simulink model "MultirotorSimPx4SeparateRotors"  (R2016b)
settings: Solver=VariableStepAuto  StartTime=0.0  StopTime=Simulation.T_END  MaxStep=Simulation.TS_MAX  RelTol=1e-3  EnableMultiTasking=on
PreLoadFcn:
  | % InitializeParameters;
undefined symbols (not defined in the file): Initial
libraries: Px4Library x19, QuaternionLibrary x12, simulink_extras x6
settings Model: Creator=jban039  LastModifiedBy=jeremie
settings DataIOCC: Decimation=10  ReturnWorkspaceOutputs=on  OutputOption=SpecifiedOutputTimes  OutputTimes=Simulation.T_OUT
settings OptimizationCC: LifeSpan=inf
settings DebuggingCC: ReadBeforeWriteMsg=DisableAll  WriteAfterWriteMsg=DisableAll  WriteAfterReadMsg=DisableAll  MultiTaskDSMMsg=none  UnconnectedLineMsg=none  AllowSymbolicDim=off  SFUnexpectedBacktrackingDiag=warning  SFNoUnconditionalDefaultTransitionDiag=warning  SFExecutionAtInitializationDiag=none
settings ModelReferenceCC: UpdateModelReferenceTargets=IfOutOfDate  ModelReferenceMinAlgLoopOccurrences=on  PropagateSignalLabelsOutOfModel=off
settings SFSimCC: SFSimEcho=off
settings GRTTargetCC: TargetLangStandard=C89/C90 (ANSI)
settings ConfigComp: CovMetricSettings=dw  CovHtmlReporting=on  CovSaveCumulativeToWorkspaceVar=on  CovSaveSingleToWorkspaceVar=on  CovExternalEMLEnable=off

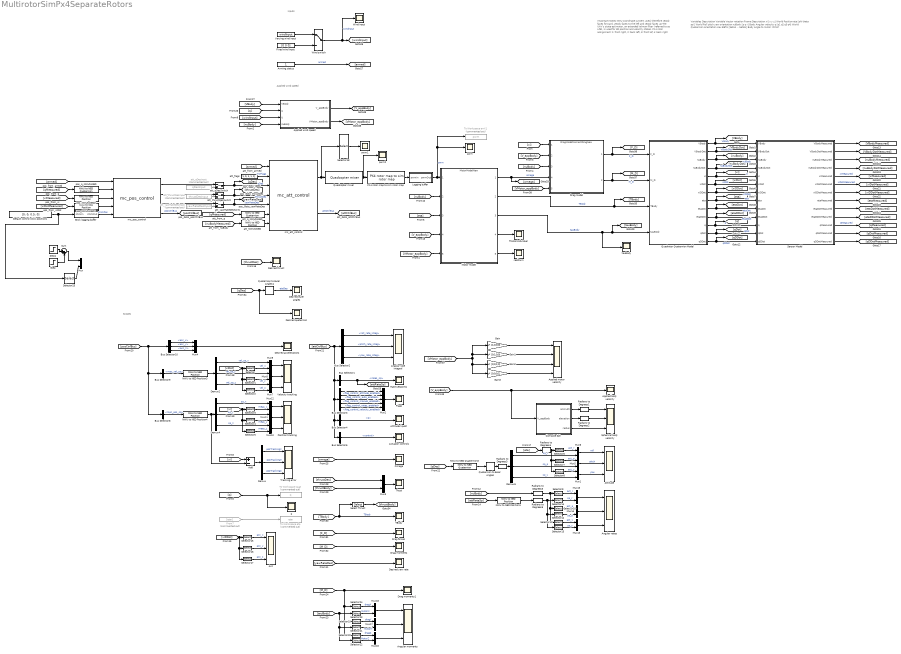
== system MultirotorSimPx4SeparateRotors ==
  note: Important Notes
      |
      | NWU coordinate system used, therefore xBody faces forward, yBody faces to the left and xBody faces up
      | The UAV's state estimator, an extended kalman filter (referred to as LPE), is used for 3D position and velocity states.
      | PX4 rotor assignment: 1: front right, 2: back left, 3: front lef, 4: back right
  note: Variables Description
      |
      | Variable
      | Vector notation
      | Frame
      | Description
      |
      | xi
      | [x y z]
      | World
      | Position
      |
      | eta
      | [phi theta psi]
      | World
      | Roll pitch yaw orientation
      |
      | nuBody
      | [p q r]
      | Body
      | Angular velocity
      |
      | q
      | [q1 q2 q3 q4]
      | World
      | Quaternion orientation
      |
      | Uav.BETA
      | [beta1 ... betaN]
      | Body
      | Angle to motor (CCW)
  note: Applied wind speed
  note: Inputs
  note: Scopes
  Acc : Scope  NumInputPorts=3
  Actuator controls : Scope
  Add : Sum  Inputs=+-
  Angular moments : Scope  NumInputPorts=3
  Angular rate integral : Scope  NumInputPorts=3
  Angular rates : Scope  NumInputPorts=3
  Applied body velocity : Scope
  Applied motor velocity : Scope  NumInputPorts=4
  Applied wind speed : Subsystem
  Arming status : Constant
  Attitude : Scope  NumInputPorts=3
  Attitude (quat) : Scope
  Bus Selector1 : BusSelector  OutputSignals=rates_sp
  Bus Selector10 : BusSelector  OutputSignals=mpc_local_pos_sp.acc_x,mpc_local_pos_sp.acc_y,mpc_local_pos_sp.acc_z
  Bus Selector2 : BusSelector  OutputSignals=controller_status.roll_rate_integ,controller_status.pitch_rate_integ,controller_status.yaw_rate_integ
  Bus Selector3 : BusSelector  OutputSignals=v_control_mode.flag_control_attitude_enabled,v_control_mode.flag_control_auto_enabled,v_control_mode.flag_control_manual_enabled,v_control_mode.flag_control_rates_enabled,v_control_mode.flag_control_velocity_enabled
  Bus Selector4 : BusSelector  OutputSignals=ctrl_state.q
  Bus Selector6 : BusSelector  OutputSignals=actuators.control
  Bus Selector8 : BusSelector  OutputSignals=mpc_pos_sp
  Bus Selector9 : BusSelector  OutputSignals=mpc_vel_sp
  Compute Sph : MATLAB Function  TreatAsAtomicUnit=on
  Default control stick positions : Constant  Value=[0; 0; 0.5; 0]
  Demux{,2,4,6} (4 alike) : Demux  Outputs=3
  Desired accelerations : Scope
  Desired euler angles : Scope
  Desired quaternion : Scope
  Desired thrust : Scope
  Desired yaw rate : Scope
  Drag forces : Scope
  Drag model : ModelReference  ModelNameDialog=DragModelMomentDragNew  SimulationMode=Normal  ModelReferenceVersion=1.250
  Drag moments : Scope
  Drag moments1 : Scope
  Fixed wind input : Constant  Value=[0 0 0]
  Flags : Scope
  From7 : From  Commented=on  GotoTag=eta
  Gain : Gain  Gain=[1;0;0;0]  Multiplication=Matrix(u*K)
  Gain1 : Gain  Gain=[0;1;0;0]  Multiplication=Matrix(u*K)
  Gain2 : Gain  Gain=[0;0;1;0]  Multiplication=Matrix(u*K)
  Gain3 : Gain  Gain=[0;0;0;1]  Multiplication=Matrix(u*K)
  Logging buffer : Subsystem
  Motor model : ModelReference  ModelNameDialog=MotorModelNew  SimulationMode=Normal  ModelReferenceVersion=1.289
  Mux{,1,3,5..18} (17 alike) : Mux  Inputs=2
  Mux2 : Mux  Inputs=5
  Mux4 : Mux  Inputs=3
  NWU to NED Position1 : Px4Library/NWU to NED Position
  NWU to NED Position3 : Px4Library/NWU to NED Position
  NWU to NED Position4 : Px4Library/NWU to NED Position
  NWU to NED Quaternion3 : Px4Library/NWU to NED Quaternion
  Omega : Scope
  PX4 rotor map to sim rotor map : Px4Library/PX4 rotor map to sim rotor map  SystemSampleTime=-1
  Position tracking : Scope  NumInputPorts=3
  Quadcopter mixer : Px4Library/Quadcopter mixer  MC_SAMPLING_PERIOD=0.002
  Quadrotor Quaternion Model : Subsystem
  Quaternion to Euler Angles : QuaternionLibrary/Quaternion to Euler Angles
  Quaternion to Euler Angles1 : QuaternionLibrary/Quaternion to Euler Angles
  Radians to Degrees{1..6} (6 alike) : simulink_extras/Transformations/Radians to Degrees
  Rate setpoints : Scope
  Select Thrust : Selector  InputPortWidth=3  IndexOptions=Index vector (dialog)  Indices=[3]  OutputSizes=1
  Selector{,3,6,9,14..15,23..24} (8 alike) : Selector  InputPortWidth=3  IndexOptions=Index vector (dialog)  Indices=1  OutputSizes=1
  Selector{1,4,7,10,12,16,19,21} (8 alike) : Selector  InputPortWidth=3  IndexOptions=Index vector (dialog)  Indices=2  OutputSizes=1
  Selector{2,5,8,11,13,17,20,22} (8 alike) : Selector  InputPortWidth=3  IndexOptions=Index vector (dialog)  Indices=3  OutputSizes=1
  Selector18 : Selector  InputPortWidth=8  IndexOptions=Index vector (dialog)  Indices=[1 2 3]  OutputSizes=1
  Selector25 : Selector  InputPortWidth=4  IndexOptions=Index vector (dialog)  Indices=[ 2 3 4 ]  OutputSizes=1
  Sensor Model : Subsystem
  Spherical body velocity : Scope  NumInputPorts=3
  Step : Step  Time=100  After=0.2  SampleTime=0
  Step1 : Step  Time=105  After=-0.2  SampleTime=0
  Stick logging buffer : Subsystem
  Sum : Sum  Inputs=|++
  TBody : Scope
  TMotorIndividual : Scope
  Thust : Scope
  To Workspace errX1 : ToWorkspace  Commented=on  VariableName=pwm  SampleTime=0.01
      settings: Save2DSignal=2-D array (concatenate along first dimension)
  To Workspace eta : ToWorkspace  Commented=on  VariableName=eta  SaveFormat=Structure With Time  SampleTime=0.01
  To Workspace quat : ToWorkspace  Commented=on  VariableName=q  SaveFormat=Structure With Time  SampleTime=0.01
  Tracking error : Scope  NumInputPorts=3
  Varying wind input : FromWorkspace  VariableName=windInput  SampleTime=0
  Velocity tracking : Scope  NumInputPorts=3
  Wind Input : Scope
  Wind switch : ManualSwitch
  att_NWUtoNED : Px4Library/NWU to NED Position
  att_flags : Constant  Value=[1, 0, 1, 1, 1]
  att_qDesInput : FromWorkspace  Commented=on  VariableName=qDesInput  SampleTime=0  Interpolate=off  OutputAfterFinalValue=Holding final value
  att_qDesSwitch : ManualSwitch
  att_q_NWUtoNED : Px4Library/NWU to NED Quaternion
  att_thrustDesInput : FromWorkspace  Commented=on  VariableName=thrustDesInput  SampleTime=0  Interpolate=off  OutputAfterFinalValue=Holding final value
  att_thrustDesSwitch : ManualSwitch
  att_yawRateDesInput : FromWorkspace  Commented=on  VariableName=yawRateDesInput  SampleTime=0  Interpolate=off  OutputAfterFinalValue=Holding final value
  att_yawRateDesSwitch : ManualSwitch
  mc_att_control : Px4Library/mc_att_control  MC_SAMPLING_PERIOD=0.004  MC_ROLL_TC=0.2  MC_PITCH_TC=0.2  MC_ROLL_P=6.5  MC_ROLLRATE_P=0.15  MC_ROLLRATE_I=0.05  MC_ROLLRATE_D=0.003  MC_ROLLRATE_FF=0.0  MC_PITCH_P=6.5  MC_PITCHRATE_P=0.15  MC_PITCHRATE_I=0.05  MC_PITCHRATE_D=0.003  MC_PITCHRATE_FF=0.0  MC_YAW_P=2.8  MC_YAWRATE_P=0.2  MC_YAWRATE_I=0.1  MC_YAWRATE_D=0.0  MC_YAWRATE_FF=0.0  MC_YAW_FF=0.5  MC_ROLLRATE_MAX=220.0  MC_PITCHRATE_MAX=220.0  MC_YAWRATE_MAX=200.0  MC_YAWRAUTO_MAX=45.0  MC_ACRO_R_MAX=360.0  MC_ACRO_P_MAX=360.0  MC_ACRO_Y_MAX=360.0  MC_RATT_TH=1.0  MC_TPA_BREAK=1.0  MC_TPA_SLOPE=1.0  VT_OPT_RECOV_EN=0.0  VT_WV_YAWR_SCL=0.15  MC_RR_INT_LIM=0.30  MC_PR_INT_LIM=0.30  MC_TPA_BREAK_P=1.0  MC_TPA_BREAK_I=1.0  MC_TPA_BREAK_D=1.0  MC_TPA_RATE_P=0.0  MC_TPA_RATE_I=0.0  MC_TPA_RATE_D=0.0  VT_TYPE=2  MC_BAT_SCALE_EN=0  MC_YR_INT_LIM=0.30
  mc_pos_control : Px4Library/mc_pos_control  THROTTLE_HOVER=Uav.THROTTLE_HOVER  MPC_SAMPLING_PERIOD=0.02  MPC_THR_MIN=0.120  MPC_THR_HOVER=0.500  MPC_ALTCTL_DZ=0.100  MPC_ALTCTL_DY=0.0  MPC_THR_MAX=0.900  MPC_MANTHR_MIN=0.080  MPC_MANTHR_MAX=0.900  MPC_Z_P=1.000  MPC_Z_VEL_P=0.200  MPC_Z_VEL_I=0.020  MPC_Z_VEL_D=0.0  MPC_Z_VEL_MAX_UP=3.0  MPC_Z_VEL_MAX=1.000  MPC_Z_VEL_MAX_DN=1.000  MPC_Z_FF=0.500  MPC_XY_P=0.950  MPC_XY_VEL_P=0.090  MPC_XY_VEL_I=0.020  MPC_XY_VEL_D=0.010  MPC_XY_CRUISE=5.0  MPC_XY_VEL_MAX=8.0  MPC_XY_FF=0.500  MPC_TILTMAX_AIR=45.0  MPC_TILTMAX_LND=12.0  MPC_LAND_SPEED=0.500  MPC_TKO_SPEED=1.500  MPC_MAN_R_MAX=35.0  MPC_MAN_P_MAX=35.0  MPC_MAN_Y_MAX=200.0  MPC_HOLD_XY_DZ=0.100  MPC_HOLD_MAX_XY=0.800  MPC_HOLD_MAX_Z=0.600  MPC_VELD_LP=5.0  MPC_ACC_HOR_MAX=5.0  MPC_ALT_MODE=0.0  MC_YAWRATE_MAX=200.0  MC_YAW_P=2.8  VT_OPT_RECOV_EN=0.0
  pos_NWUtoNED1 : Px4Library/NWU to NED Position
  pos_NWUtoNED2 : Px4Library/NWU to NED Position
  pos_q_NWUtoNED : Px4Library/NWU to NED Quaternion
  pwm : Scope
  pwm1 : Scope
  pwm2 : Scope
  q : Scope
  realPwm : Scope
  tauBody : Scope
  wires:
  Motor model/1 -> [omega], Drag model/4  "omega"
  Motor model/2 -> [TBody], Quadrotor Quaternion Model/3(TBody)  "TBody"
  Drag model/2 -> [M_D], Quadrotor Quaternion Model/2(M_D)  "M_D"
  Quadrotor Quaternion Model/1(VBody) -> Sensor Model/1(VBody), [VBody]  "VBody"
  Quadrotor Quaternion Model/2(VBodyDot) -> Sensor Model/2(VBodyDot), [VBodyDot]  "VBodyDot"
  Quadrotor Quaternion Model/3(nuBody) -> Sensor Model/3(nuBody), [nuBody]  "nuBody"
  Quadrotor Quaternion Model/4(nuBodyDot) -> Sensor Model/4(nuBodyDot), [nuBodyDot]  "nuBodyDot"
  Quadrotor Quaternion Model/5(xi) -> Sensor Model/5(xi), [xi]  "xi"
  Quadrotor Quaternion Model/6(xiDot) -> Sensor Model/6(xiDot), [xiDot]  "xiDot"
  Quadrotor Quaternion Model/7(xiDDot) -> Sensor Model/7(xiDDot), [xiDDot]  "xiDDot"
  Quadrotor Quaternion Model/8(eta) -> Sensor Model/8(eta), [eta]  "eta"
  Quadrotor Quaternion Model/9(etaDot) -> Sensor Model/9(etaDot), [etaDot]  "etaDot"
  Quadrotor Quaternion Model/10(etaDDot) -> Sensor Model/10(etaDDot), [etaDDot]  "etaDDot"
  [V_appBody] -> Drag model/2
  [nuBody] -> Motor model/2
  Quadrotor Quaternion Model/11(q) -> Sensor Model/11(q), [q]  "q"
  Quadrotor Quaternion Model/12(qDot) -> Sensor Model/12(qDot), [qDot]  "qDot"
  Quadrotor Quaternion Model/13(qDDot) -> Sensor Model/13(qDDot), [qDDot]  "qDDot"
  Drag model/1 -> Quadrotor Quaternion Model/1(F_D), [F_D]  "F_D"
  Sensor Model/1(VBodyMeasured) -> [VBodyMeasured]
  Sensor Model/2(VBodyDotMeasured) -> [VBodyDotMeasured]
  Sensor Model/3(nuBodyMeasured) -> [nuBodyMeasured]
  Sensor Model/4(nuBodyDotMeasured) -> [nuBodyDotMeasured]
  Sensor Model/5(xiMeasured) -> [xiMeasured]  "xiMeasured"
  Sensor Model/6(xiDotMeasured) -> [xiDotMeasured]  "xiDotMeasured"
  Sensor Model/7(xiDDotMeasured) -> [xiDDotMeasured]
  Sensor Model/8(etaMeasured) -> [etaMeasured]
  Sensor Model/9(etaDotMeasured) -> [etaDotMeasured]
  Sensor Model/10(etaDDotMeasured) -> [etaDDotMeasured]
  Sensor Model/11(qMeasured) -> [qMeasured]  "qMeasured"
  Sensor Model/12(qDotMeasured) -> [qDotMeasured]
  Sensor Model/13(qDDotMeasured) -> [qDDotMeasured]
  Logging buffer/1(pwmOut) -> To Workspace errX1/1, pwm/1, Motor model/1  "pwm"
  [nuBodyMeasured] -> att_NWUtoNED/1
  Bus Selector2/1 -> Angular rate integral/1  "<roll_rate_integ>"
  Bus Selector2/2 -> Angular rate integral/2  "<pitch_rate_integ>"
  Bus Selector2/3 -> Angular rate integral/3  "<yaw_rate_integ>"
  [attCtrlBus] -> Bus Selector2/1, Bus Selector1/1, Bus Selector6/1, Bus Selector4/1, Bus Selector3/1
  Bus Selector1/1 -> [attRateSp], Rate setpoints/1  "<rates_sp>"
  Bus Selector3/1 -> Mux2/1  "<flag_control_attitude_enabled>"
  Bus Selector3/2 -> Mux2/2  "<flag_control_auto_enabled>"
  Bus Selector3/3 -> Mux2/3  "<flag_control_manual_enabled>"
  Bus Selector3/4 -> Mux2/4  "<flag_control_rates_enabled>"
  Bus Selector3/5 -> Mux2/5  "<flag_control_velocity_enabled>"
  Mux2/1 -> Flags/1
  Bus Selector4/1 -> Attitude (quat)/1  "<q>"
  Bus Selector6/1 -> Actuator controls/1  "<control>"
  mc_pos_control/1 -> att_qDesSwitch/1
  [posCtrlBus] -> Bus Selector10/1, Bus Selector9/1, Bus Selector8/1
  [qMeasured] -> pos_q_NWUtoNED/1
  Stick logging buffer/1(stickOut) -> mc_pos_control/5  "stickPos"
  [qMeasured] -> att_q_NWUtoNED/1
  att_q_NWUtoNED/1 -> mc_att_control/6
  att_NWUtoNED/1 -> mc_att_control/7
  pos_q_NWUtoNED/1 -> mc_pos_control/2
  mc_pos_control/3 -> att_yawRateDesSwitch/1
  mc_pos_control/2 -> att_thrustDesSwitch/1
  Bus Selector9/1 -> NWU to NED Position3/1  "<mpc_vel_sp>"
  pos_NWUtoNED1/1 -> mc_pos_control/4
  pos_NWUtoNED2/1 -> mc_pos_control/3
  [xiMeasured] -> pos_NWUtoNED2/1
  Bus Selector10/1 -> Mux4/1  "<acc_x>"
  Bus Selector10/2 -> Mux4/2  "<acc_y>"
  Bus Selector10/3 -> Mux4/3  "<acc_z>"
  Mux4/1 -> Desired accelerations/1
  Selector6/1 -> Mux6/1  "act_r"
  Selector7/1 -> Mux5/1  "act_p"
  Mux7/1 -> Velocity tracking/3
  Mux8/1 -> Velocity tracking/2
  Mux9/1 -> Velocity tracking/1
  Demux2/1 -> Mux9/1  "vel_sp_x"
  Selector/1 -> Mux9/2  "vel_x"
  Demux2/2 -> Mux8/1  "vel_sp_y"
  Selector1/1 -> Mux8/2  "vel_y"
  Demux2/3 -> Mux7/1  "vel_sp_z"
  Selector2/1 -> Mux7/2  "vel_z"
  Mux10/1 -> Position tracking/3
  Mux11/1 -> Position tracking/2
  Mux12/1 -> Position tracking/1
  Demux4/1 -> Mux12/1  "sp_x"
  Selector3/1 -> Mux12/2  "meas_x"
  Demux4/2 -> Mux11/1  "sp_y"
  Selector4/1 -> Mux11/2  "meas_y"
  Demux4/3 -> Mux10/1  "sp_z"
  Selector5/1 -> Mux10/2  "meas_z"
  Quaternion to Euler Angles/1 -> Radians to Degrees3/1
  Demux6/1 -> Mux6/2  "sp_r"
  Demux6/2 -> Mux5/2  "sp_p"
  Demux6/3 -> Mux1/2  "sp_y"
  Selector8/1 -> Mux1/1  "act_y"
  NWU to NED Quaternion3/1 -> Quaternion to Euler Angles/1
  mc_att_control/1 -> Selector18/1, Quadcopter mixer/1
  Quadcopter mixer/1 -> pwm2/1, PX4 rotor map to sim rotor map/1
  PX4 rotor map to sim rotor map/1 -> Logging buffer/1(pwmIn)
  Bus Selector8/1 -> NWU to NED Position4/1  "<mpc_pos_sp>"
  NWU to NED Position3/1 -> Demux2/1
  NWU to NED Position4/1 -> Add/2, Demux4/1
  Add/1 -> Demux/1
  Demux/1 -> Tracking error/1  "posTrackingX"
  Demux/2 -> Tracking error/2  "posTrackingY"
  Demux/3 -> Tracking error/3  "posTrackingZ"
  [nuBody] -> Drag model/3
  Mux6/1 -> Attitude/1  "roll"
  Mux5/1 -> Attitude/2  "pitch"
  [eta] -> Motor model/3
  [q] -> q/1, To Workspace quat/1
  From7/1 -> To Workspace eta/1
  [xiDot] -> Selector2/1, Selector1/1, Selector/1
  [xi] -> Selector5/1, Selector4/1, Selector3/1
  [xi] -> Add/1
  Wind switch/1 -> Wind Input/1, [windInput]  "windInput"
  [V_appBody] -> Motor model/4
  att_flags/1 -> mc_att_control/2  "mcFlags"
  Arming status/1 -> [armed]  "armed"
  mc_pos_control/4 -> [posCtrlBus]  "posCtrlBus"
  mc_att_control/2 -> [attCtrlBus]  "attCtrlBus"
  [qDes] -> NWU to NED Quaternion3/1
  [armed] -> mc_att_control/1
  [armed] -> mc_pos_control/1
  Fixed wind input/1 -> Wind switch/2
  Varying wind input/1 -> Wind switch/1
  [omega] -> Omega/1
  Radians to Degrees3/1 -> Demux6/1
  Radians to Degrees4/1 -> Selector8/1, Selector7/1, Selector6/1
  [eta] -> Radians to Degrees4/1
  Motor model/4 -> TMotorIndividual/1
  [thrustDes] -> Mux3/1
  [thrustBody] -> Mux3/2
  Mux3/1 -> Thust/1
  Motor model/5 -> realPwm/1
  [xi] -> Drag model/1
  [xiDotMeasured] -> pos_NWUtoNED1/1
  [TBody] -> Select Thrust/1, TBody/1  "TBody"
  Select Thrust/1 -> [thrustBody]
  [F_D] -> Drag forces/1
  [V_appBody] -> Compute Sph/1(V_appBody), Applied body velocity/1
  Compute Sph/1(azimuth) -> Radians to Degrees1/1
  Compute Sph/2(elevation) -> Radians to Degrees2/1
  Compute Sph/3(radius) -> Spherical body velocity/3
  Radians to Degrees1/1 -> Spherical body velocity/1
  Radians to Degrees2/1 -> Spherical body velocity/2
  [M_D] -> Drag moments/1
  [VMotor_appBody] -> Motor model/5
  [VMotor_appBody] -> Gain3/1, Gain2/1, Gain/1, Gain1/1
  Gain/1 -> Applied motor velocity/1
  Gain1/1 -> Applied motor velocity/2
  Gain2/1 -> Applied motor velocity/3
  Gain3/1 -> Applied motor velocity/4
  [VMotor_appBody] -> Drag model/5
  att_qDesSwitch/1 -> [qDes], mc_att_control/3  "qDes"
  att_thrustDesSwitch/1 -> [thrustDes], mc_att_control/4  "thrustDes"
  att_yawRateDesSwitch/1 -> [yawRateDes], mc_att_control/5  "yawRateDes"
  att_yawRateDesInput/1 -> att_yawRateDesSwitch/2
  att_thrustDesInput/1 -> att_thrustDesSwitch/2
  att_qDesInput/1 -> att_qDesSwitch/2
  [yawRateDes] -> Desired yaw rate/1
  Mux1/1 -> Attitude/3  "yaw"
  Motor model/3 -> tauBody/1, [tauBody], Quadrotor Quaternion Model/4(tauBody)  "tauBody"
  [VBody] -> Applied wind speed/1(VBody)
  [q] -> Applied wind speed/2(q)
  [windInput] -> Applied wind speed/3(U)
  Applied wind speed/1(V_appBody) -> [V_appBody]
  Applied wind speed/2(VMotor_appBody) -> [VMotor_appBody]
  [nuBody] -> Applied wind speed/4(nuBody)
  Selector9/1 -> Mux15/1  "act_r"
  Selector10/1 -> Mux14/1  "act_p"
  Selector11/1 -> Mux13/1  "act_y"
  Mux15/1 -> Angular rates/1
  Mux14/1 -> Angular rates/2
  Radians to Degrees5/1 -> Selector9/1, Selector11/1, Selector10/1
  [nuBody] -> Radians to Degrees5/1
  Mux13/1 -> Angular rates/3
  Radians to Degrees6/1 -> Selector14/1, Selector13/1, Selector12/1
  Selector14/1 -> Mux15/2  "sp_r"
  Selector12/1 -> Mux14/2  "sp_p"
  Selector13/1 -> Mux13/2  "sp_y"
  [attRateSp] -> NWU to NED Position1/1
  NWU to NED Position1/1 -> Radians to Degrees6/1
  Selector15/1 -> Acc/1  "acc_x"
  Selector16/1 -> Acc/2  "acc_y"
  Selector17/1 -> Acc/3  "acc_z"
  [xiDDot] -> Selector15/1, Selector16/1, Selector17/1
  [thrustDes] -> Desired thrust/1
  Selector18/1 -> pwm1/1
  [M_D] -> Selector20/1, Selector19/1, Selector24/1, Drag moments1/1
  Mux18/1 -> Angular moments/1
  Mux17/1 -> Angular moments/2
  Mux16/1 -> Angular moments/3
  Selector24/1 -> Mux18/1  "dragX"
  Selector23/1 -> Mux18/2  "motorX"
  Selector19/1 -> Mux17/1  "dragY"
  Selector21/1 -> Mux17/2  "motorY"
  Selector20/1 -> Mux16/1  "dragZ"
  Selector22/1 -> Mux16/2  "MotorZ"
  [tauBody] -> Selector22/1, Selector21/1, Selector23/1
  Default control stick positions/1 -> Stick logging buffer/1(stickIn), Selector25/1
  [qDes] -> Desired quaternion/1, Quaternion to Euler Angles1/1
  Quaternion to Euler Angles1/1 -> Desired euler angles/1  "etaDes"
  Sum/1 -> Mux/1
  Selector25/1 -> Mux/2
  Step1/1 -> Sum/1
  Step/1 -> Sum/2

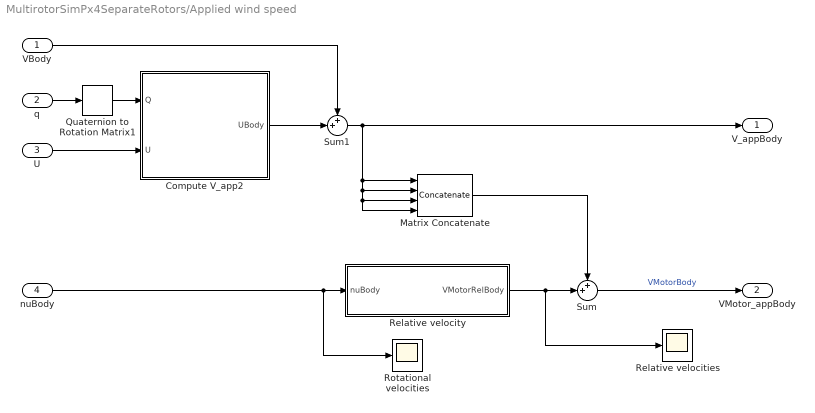
== system MultirotorSimPx4SeparateRotors/Applied wind speed ==
  VBody : Inport  Unit=m/s
  q : Inport  Port=2
  U : Inport  Port=3  Unit=m/s
  nuBody : Inport  Port=4  Unit=rad/s
  Compute V_app2 : MATLAB Function  TreatAsAtomicUnit=on
  Matrix Concatenate : Concatenate  NumInputs=4  Mode=Multidimensional array  ConcatenateDimension=2
  Quaternion to Rotation Matrix1 : QuaternionLibrary/Quaternion to Rotation Matrix
  Relative velocities : Scope
  Relative velocity : MATLAB Function  TreatAsAtomicUnit=on
  Rotational velocities : Scope
  Sum : Sum  Inputs=++|
  Sum1 : Sum  Inputs=++|
  V_appBody : Outport  Unit=m/s
  VMotor_appBody : Outport  Port=2  Unit=m/s
  wires:
  U/1 -> Compute V_app2/2(U)
  Sum/1 -> VMotor_appBody/1  "VMotorBody"
  Quaternion to Rotation Matrix1/1 -> Compute V_app2/1(Q)
  nuBody/1 -> Rotational velocities/1, Relative velocity/1(nuBody)
  Matrix Concatenate/1 -> Sum/1
  VBody/1 -> Sum1/1
  q/1 -> Quaternion to Rotation Matrix1/1
  Relative velocity/1(VMotorRelBody) -> Relative velocities/1, Sum/2
  Compute V_app2/1(UBody) -> Sum1/2
  Sum1/1 -> V_appBody/1, Matrix Concatenate/4, Matrix Concatenate/3, Matrix Concatenate/2, Matrix Concatenate/1

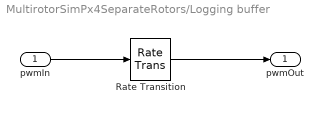
== system MultirotorSimPx4SeparateRotors/Logging buffer ==
  pwmIn : Inport
  Rate Transition : RateTransition
  pwmOut : Outport
  wires:
  pwmIn/1 -> Rate Transition/1
  Rate Transition/1 -> pwmOut/1

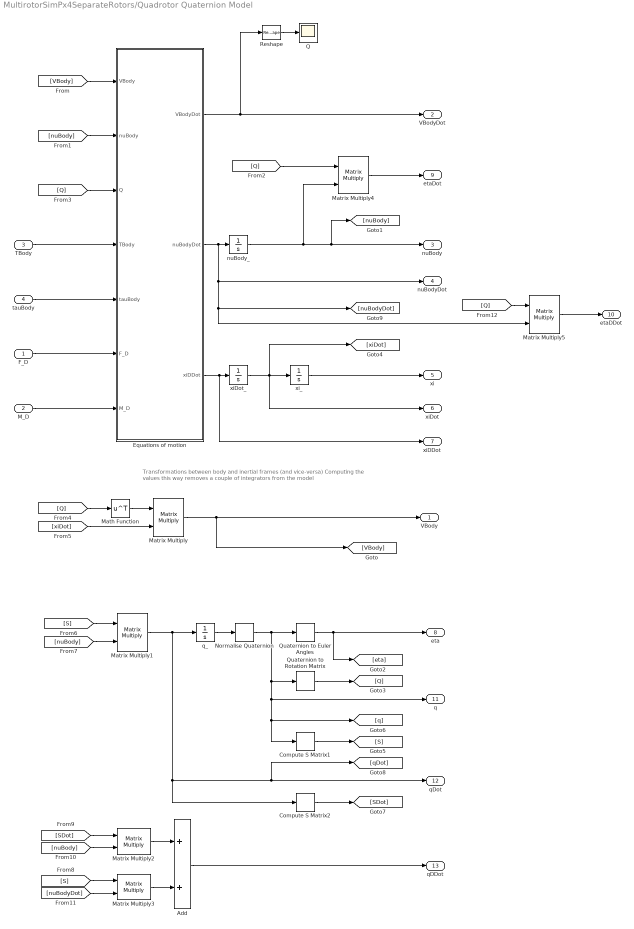
== system MultirotorSimPx4SeparateRotors/Quadrotor Quaternion Model ==
  note: Transformations between body and inertial frames (and vice-versa)
      | Computing the values this way removes a couple of integrators from the model
  F_D : Inport  Unit=N
  M_D : Inport  Port=2  Unit=N*m
  TBody : Inport  Port=3  Unit=N
  tauBody : Inport  Port=4  Unit=N*m
  Add : Sum
  Compute S Matrix1 : QuaternionLibrary/Compute S Matrix
  Compute S Matrix2 : QuaternionLibrary/Compute S Matrix
  Equations of motion : MATLAB Function  TreatAsAtomicUnit=on
  Math Function : Math  Operator=transpose  SaturateOnIntegerOverflow=on
  Matrix Multiply{,1..5} (6 alike) : Product  Multiplication=Matrix(*)
  Normalise Quaternion : QuaternionLibrary/Normalise Quaternion
  Q : Scope
  Quaternion to Euler Angles : QuaternionLibrary/Quaternion to Euler Angles
  Quaternion to Rotation Matrix : QuaternionLibrary/Quaternion to Rotation Matrix
  Reshape : Reshape  OutputDimensionality=Column vector (2-D)
  nuBody_ : Integrator  InitialCondition=Initial.NU_BODY
  q_ : Integrator  InitialCondition=Initial.Q
  xiDot_ : Integrator  InitialCondition=Initial.XI_DOT
  xi_ : Integrator  InitialCondition=Initial.XI
  VBody : Outport  Unit=m/s
  VBodyDot : Outport  Port=2  Unit=m/s^2
  nuBody : Outport  Port=3  Unit=rad/s
  nuBodyDot : Outport  Port=4  Unit=rad/s^2
  xi : Outport  Port=5  Unit=m
  xiDot : Outport  Port=6  Unit=m/s
  xiDDot : Outport  Port=7  Unit=m/s^2
  eta : Outport  Port=8  Unit=rad
  etaDot : Outport  Port=9  Unit=rad/s
  etaDDot : Outport  Port=10  Unit=rad/s^2
  q : Outport  Port=11
  qDot : Outport  Port=12
  qDDot : Outport  Port=13
  wires:
  Equations of motion/1(VBodyDot) -> Reshape/1, VBodyDot/1
  xi_/1 -> xi/1
  [nuBody] -> Equations of motion/2(nuBody)
  [VBody] -> Equations of motion/1(VBody)
  tauBody/1 -> Equations of motion/5(tauBody)
  TBody/1 -> Equations of motion/4(TBody)
  Equations of motion/3(xiDDot) -> xiDot_/1, xiDDot/1
  F_D/1 -> Equations of motion/6(F_D)
  Matrix Multiply/1 -> VBody/1, [VBody]
  M_D/1 -> Equations of motion/7(M_D)
  nuBody_/1 -> Matrix Multiply4/2, [nuBody], nuBody/1
  Equations of motion/2(nuBodyDot) -> nuBody_/1, nuBodyDot/1, Matrix Multiply5/2, [nuBodyDot]
  q_/1 -> Normalise Quaternion/1
  Quaternion to Euler Angles/1 -> eta/1, [eta]
  Matrix Multiply4/1 -> etaDot/1
  Quaternion to Rotation Matrix/1 -> [Q]
  [Q] -> Equations of motion/3(Q)
  [Q] -> Math Function/1
  [xiDot] -> Matrix Multiply/2
  Math Function/1 -> Matrix Multiply/1
  [S] -> Matrix Multiply1/1
  [nuBody] -> Matrix Multiply1/2
  Compute S Matrix2/1 -> [SDot]
  [S] -> Matrix Multiply3/1
  Matrix Multiply1/1 -> qDot/1, [qDot], Compute S Matrix2/1, q_/1
  [SDot] -> Matrix Multiply2/1
  [nuBody] -> Matrix Multiply2/2
  [nuBodyDot] -> Matrix Multiply3/2
  Matrix Multiply2/1 -> Add/1
  Matrix Multiply3/1 -> Add/2
  Normalise Quaternion/1 -> Quaternion to Euler Angles/1, q/1, Compute S Matrix1/1, [q], Quaternion to Rotation Matrix/1
  Compute S Matrix1/1 -> [S]
  [Q] -> Matrix Multiply4/1
  Add/1 -> qDDot/1
  [Q] -> Matrix Multiply5/1
  Matrix Multiply5/1 -> etaDDot/1
  Reshape/1 -> Q/1
  xiDot_/1 -> xi_/1, [xiDot], xiDot/1

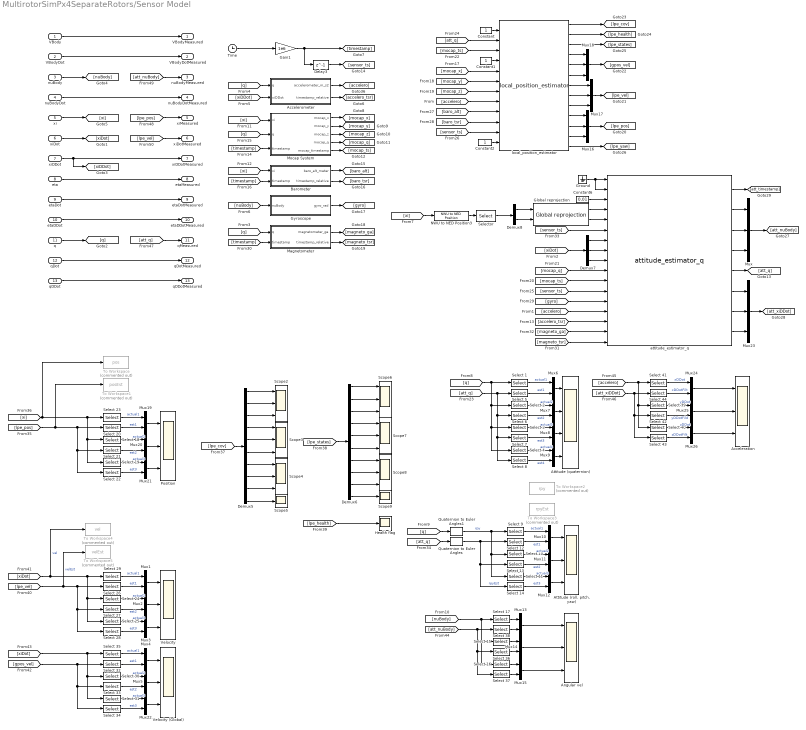
== system MultirotorSimPx4SeparateRotors/Sensor Model ==
  VBody : Inport  Unit=m/s  PortDimensions=3
  VBodyDot : Inport  Port=2  Unit=m/s^2  PortDimensions=3
  nuBody : Inport  Port=3  Unit=rad/s  PortDimensions=3
  nuBodyDot : Inport  Port=4  Unit=rad/s^2  PortDimensions=3
  xi : Inport  Port=5  Unit=m  PortDimensions=3
  xiDot : Inport  Port=6  Unit=m/s  PortDimensions=3
  xiDDot : Inport  Port=7  Unit=m/s^2  PortDimensions=3
  eta : Inport  Port=8  Unit=rad  PortDimensions=3
  etaDot : Inport  Port=9  Unit=rad/s  PortDimensions=3
  etaDDot : Inport  Port=10  Unit=rad/s^2  PortDimensions=3
  q : Inport  Port=11  PortDimensions=4
  qDot : Inport  Port=12  PortDimensions=4
  qDDot : Inport  Port=13  PortDimensions=4
  Acceleration : Scope  NumInputPorts=3
  Accelerometer : Subsystem
  Angular vel : Scope  NumInputPorts=3
  Attitude (quaternion) : Scope  NumInputPorts=4
  "Attitude (roll, pitch, yaw)" : Scope  NumInputPorts=3
  Barometer : Subsystem
  Constant : Constant
  Constant1 : Constant
  Constant2 : Constant
  Constant6 : Constant  Value=0.01
  Delay3 : Delay  DelayLength=1  SampleTime=1/400
  Demux5 : Demux  Outputs=10
  Demux6 : Demux  Outputs=10
  Demux7 : Demux  Outputs=3
  Demux8 : Demux  Outputs=2
  Gain1 : Gain  Gain=1e6
  Global reprojection : Px4Library/Global reprojection  LAT0=-36.865577  LON0=174.772065
  Ground : Ground
  Gyroscope : Subsystem
  Health flag : Scope
  Magnetometer : Subsystem
  Mocap System : Subsystem
  Mux{,16..18,23} (5 alike) : Mux  Inputs=3
  Mux{1..15,19..22,24..26} (22 alike) : Mux  Inputs=2
  NWU to NED Position3 : Px4Library/NWU to NED Position
  Position : Scope  NumInputPorts=3
  Quaternion to Euler Angles : QuaternionLibrary/Quaternion to Euler Angles
  Quaternion to Euler Angles1 : QuaternionLibrary/Quaternion to Euler Angles
  Scope{2..4,6..8} (6 alike) : Scope  NumInputPorts=3
  Scope5 : Scope
  Scope9 : Scope
  Select 1 : Selector  InputPortWidth=4  IndexOptions=Index vector (dialog)  Indices=1  OutputSizes=1
  Select {10,13,15,18,21,24,27,30,33,36,39,42} (12 alike) : Selector  InputPortWidth=3  IndexOptions=Index vector (dialog)  Indices=2  OutputSizes=1
  Select {11,14,16,19,22,25,28,31,34,37,40,43} (12 alike) : Selector  InputPortWidth=3  IndexOptions=Index vector (dialog)  Indices=3  OutputSizes=1
  Select {9,12,17,20,23,26,29,32,35,38,41,44} (12 alike) : Selector  InputPortWidth=3  IndexOptions=Index vector (dialog)  Indices=1  OutputSizes=1
  Select 2 : Selector  InputPortWidth=4  IndexOptions=Index vector (dialog)  Indices=2  OutputSizes=1
  Select 3 : Selector  InputPortWidth=4  IndexOptions=Index vector (dialog)  Indices=3  OutputSizes=1
  Select 4 : Selector  InputPortWidth=4  IndexOptions=Index vector (dialog)  Indices=4  OutputSizes=1
  Select 5 : Selector  InputPortWidth=4  IndexOptions=Index vector (dialog)  Indices=1  OutputSizes=1
  Select 6 : Selector  InputPortWidth=4  IndexOptions=Index vector (dialog)  Indices=2  OutputSizes=1
  Select 7 : Selector  InputPortWidth=4  IndexOptions=Index vector (dialog)  Indices=3  OutputSizes=1
  Select 8 : Selector  InputPortWidth=4  IndexOptions=Index vector (dialog)  Indices=4  OutputSizes=1
  Selector : Selector  InputPortWidth=3  IndexOptions=Index vector (dialog)  Indices=[1 2]  OutputSizes=1
  Time : Clock
  To Workspace : ToWorkspace  Commented=on  VariableName=pos  SaveFormat=Structure With Time  SampleTime=-1
  To Workspace1 : ToWorkspace  Commented=on  VariableName=posEst  SaveFormat=Structure With Time  SampleTime=-1
  To Workspace2 : ToWorkspace  Commented=on  VariableName=rpy  SaveFormat=Structure With Time  SampleTime=-1
  To Workspace3 : ToWorkspace  Commented=on  VariableName=rpyEst  SaveFormat=Structure With Time  SampleTime=-1
  To Workspace4 : ToWorkspace  Commented=on  VariableName=vel  SaveFormat=Structure With Time  SampleTime=-1
  To Workspace5 : ToWorkspace  Commented=on  VariableName=velEst  SaveFormat=Structure With Time  SampleTime=-1
  Velocity : Scope  NumInputPorts=3
  Velocity (Global) : Scope  NumInputPorts=3
  attitude_estimator_q : Px4Library/attitude_estimator_q  Q_SAMPLING_PERIOD=1/250  INIT_Q="[1  0  0  0]"  ATT_W_ACC=0.2  ATT_W_MAG=0.1  ATT_W_EXT_HDG=0.1  ATT_W_GYRO_BIAS=0.1  ATT_MAG_DECL=0.0  ATT_MAG_DECL_A=1  ATT_EXT_HDG_M=2  ATT_ACC_COMP=1  ATT_BIAS_MAX=0.05  FW_ARSP_MODE=0
  local_position_estimator : Px4Library/local_position_estimator  LPE_SAMPLING_PERIOD=0.01  LPE_ACC_XY=0.012  LPE_ACC_Z=0.02  LPE_BAR_Z=3  LPE_EPH_MAX=3  LPE_EPV_MAX=5  LPE_FAKE_ORIGIN=0  LPE_FGYRO_HP=0.001  LPE_FLW_OFF_Z=0  LPE_FLW_QMIN=150  LPE_FLW_R=7  LPE_FLW_RR=7  LPE_FLW_SCALE=1.3  LPE_GPS_DELAY=0.29  LPE_GPS_VXY=0.25  LPE_GPS_VZ=0.25  LPE_GPS_XY=1  LPE_GPS_Z=3  LPE_LAND_VXY=0.05  LPE_LAND_Z=0.03  LPE_LAT=47.3977  LPE_LDR_OFF_Z=0  LPE_LDR_Z=0.03  LPE_LON=8.5456  LPE_PN_B=0.001  LPE_PN_P=0.1  LPE_PN_T=0.001  LPE_PN_V=0.1  LPE_SNR_OFF_Z=0  LPE_SNR_Z=0.05  LPE_T_MAX_GRADE=1  LPE_VIC_P=0.001  LPE_VIS_DELAY=0.1  LPE_VIS_XY=0.1  LPE_VIS_Z=0.5  LPE_VXY_PUB=0.3  LPE_X_LP=5  LPE_Z_PUB=1  LPE_FUSION=193  Barometer=on  GPS=off  LIDAR=off  Flow=off  Sonar=off  Vision=off  Mocap=on  Land=on
  VBodyMeasured : Outport  Unit=m/s
  VBodyDotMeasured : Outport  Port=2  Unit=m/s^2
  nuBodyMeasured : Outport  Port=3  Unit=rad/s
  nuBodyDotMeasured : Outport  Port=4  Unit=rad/s^2
  xiMeasured : Outport  Port=5  Unit=m
  xiDotMeasured : Outport  Port=6  Unit=m/s
  xiDDotMeasured : Outport  Port=7  Unit=m/s^2
  etaMeasured : Outport  Port=8  Unit=rad
  etaDotMeasured : Outport  Port=9  Unit=rad/s
  etaDDotMeasured : Outport  Port=10  Unit=rad/s^2
  qMeasured : Outport  Port=11
  qDotMeasured : Outport  Port=12
  qDDotMeasured : Outport  Port=13
  wires:
  xiDot/1 -> [xiDot]
  xi/1 -> [xi]
  nuBodyDot/1 -> nuBodyDotMeasured/1
  nuBody/1 -> [nuBody]
  VBodyDot/1 -> VBodyDotMeasured/1
  VBody/1 -> VBodyMeasured/1
  eta/1 -> etaMeasured/1
  etaDot/1 -> etaDotMeasured/1
  etaDDot/1 -> etaDDotMeasured/1
  q/1 -> [q]
  qDot/1 -> qDotMeasured/1
  qDDot/1 -> qDDotMeasured/1
  [att_q] -> local_position_estimator/2
  [mocap_x] -> local_position_estimator/5
  [mocap_z] -> local_position_estimator/7
  local_position_estimator/10 -> Mux16/1
  local_position_estimator/11 -> Mux16/2
  local_position_estimator/12 -> Mux16/3
  Demux5/2 -> Scope2/2
  Demux5/1 -> Scope2/1
  Demux5/3 -> Scope2/3
  Demux5/4 -> Scope3/1
  Demux5/5 -> Scope3/2
  Demux5/6 -> Scope3/3
  Demux5/7 -> Scope4/1
  Demux5/8 -> Scope4/2
  Demux5/9 -> Scope4/3
  Demux5/10 -> Scope5/1
  [lpe_states] -> Demux6/1
  Demux6/2 -> Scope6/2
  Demux6/1 -> Scope6/1
  Demux6/3 -> Scope6/3
  Demux6/4 -> Scope7/1
  Demux6/5 -> Scope7/2
  Demux6/6 -> Scope7/3
  Demux6/7 -> Scope8/1
  Demux6/8 -> Scope8/2
  Demux6/9 -> Scope8/3
  Demux6/10 -> Scope9/1
  Constant1/1 -> local_position_estimator/4
  [lpe_health] -> Health flag/1
  Constant/1 -> local_position_estimator/1
  [mocap_ts] -> local_position_estimator/3
  [xiDot] -> Demux7/1
  Time/1 -> Gain1/1
  [accelero_tsr] -> attitude_estimator_q/15
  Global reprojection/1 -> attitude_estimator_q/4
  Global reprojection/2 -> attitude_estimator_q/5
  [xi] -> NWU to NED Position3/1
  NWU to NED Position3/1 -> Selector/1
  Selector/1 -> Demux8/1
  Demux8/1 -> Global reprojection/1
  Demux8/2 -> Global reprojection/2
  [att_q] -> Select 8/1, Select 7/1, Select 6/1, Select 5/1
  [q] -> Select 2/1, Select 3/1, Select 4/1, Select 1/1
  Mux6/1 -> Attitude (quaternion)/1
  Mux7/1 -> Attitude (quaternion)/2
  Mux8/1 -> Attitude (quaternion)/3
  Mux9/1 -> Attitude (quaternion)/4
  Select 4/1 -> Mux9/1  "actual4"
  Select 8/1 -> Mux9/2  "est4"
  Select 3/1 -> Mux8/1  "actual3"
  Select 7/1 -> Mux8/2  "est3"
  Select 6/1 -> Mux7/2  "est2"
  Select 2/1 -> Mux7/1  "actual2"
  Select 5/1 -> Mux6/2  "est1"
  Select 1/1 -> Mux6/1  "actual1"
  Constant6/1 -> attitude_estimator_q/3
  [q] -> Magnetometer/1(q)
  Mux10/1 -> "Attitude (roll, pitch, yaw)"/1
  Mux11/1 -> "Attitude (roll, pitch, yaw)"/2
  Mux12/1 -> "Attitude (roll, pitch, yaw)"/3
  Select 11/1 -> Mux12/1  "actual3"
  Select 14/1 -> Mux12/2  "est3"
  Select 13/1 -> Mux11/2  "est2"
  Select 10/1 -> Mux11/1  "actual2"
  Select 12/1 -> Mux10/2  "est1"
  Select 9/1 -> Mux10/1  "actual1"
  [q] -> Quaternion to Euler Angles1/1
  Quaternion to Euler Angles1/1 -> Select 11/1, Select 10/1, Select 9/1  "rpy"
  Quaternion to Euler Angles/1 -> Select 14/1, Select 13/1, Select 12/1  "rpyEst"
  Mux13/1 -> Angular vel/1
  Mux14/1 -> Angular vel/2
  Mux15/1 -> Angular vel/3
  Select 17/1 -> Mux13/1
  Select 15/1 -> Mux14/1
  Select 16/1 -> Mux15/1
  [nuBody] -> Select 17/1, Select 16/1, Select 15/1
  Demux7/2 -> attitude_estimator_q/8
  [accelero] -> attitude_estimator_q/14
  [sensor_ts] -> attitude_estimator_q/12
  [magneto_ga] -> attitude_estimator_q/16
  [nuBody] -> Gyroscope/1(nuBody)
  [gyro] -> attitude_estimator_q/13
  [q] -> Accelerometer/1(q)
  [xiDDot] -> Accelerometer/2(xiDDot)
  Accelerometer/1(accelerometer_m_s2) -> [accelero]
  Accelerometer/2(timestamp_relative) -> [accelero_tsr]
  [mocap_q] -> attitude_estimator_q/10
  [mocap_ts] -> attitude_estimator_q/11
  Gain1/1 -> Delay3/1, [timestamp]
  [timestamp] -> Mocap System/3(timestamp)
  [q] -> Mocap System/2(q)
  [xi] -> Mocap System/1(xi)
  Constant2/1 -> local_position_estimator/12
  [baro_alt] -> local_position_estimator/9
  [baro_tsr] -> local_position_estimator/10
  Mocap System/1(mocap_x) -> [mocap_x]
  Mocap System/2(mocap_y) -> [mocap_y]
  Mocap System/3(mocap_z) -> [mocap_z]
  [mocap_y] -> local_position_estimator/6
  Mocap System/4(mocap_q) -> [mocap_q]
  Mocap System/5(mocap_timestamp) -> [mocap_ts]
  attitude_estimator_q/5 -> [att_q]
  Delay3/1 -> [sensor_ts]
  [sensor_ts] -> local_position_estimator/11
  [xi] -> Barometer/1(xi)
  [timestamp] -> Barometer/2(timestamp)
  Barometer/1(baro_alt_meter) -> [baro_alt]
  Barometer/2(timestamp_relative) -> [baro_tsr]
  Gyroscope/1(gyro_rad) -> [gyro]
  [timestamp] -> Magnetometer/2(timestamp)
  Magnetometer/2(timestamp_relative) -> [magneto_tsr]
  Magnetometer/1(magnetometer_ga) -> [magneto_ga]
  [magneto_tsr] -> attitude_estimator_q/17
  Demux7/1 -> attitude_estimator_q/7
  Demux7/3 -> attitude_estimator_q/9
  [sensor_ts] -> attitude_estimator_q/6
  Mux16/1 -> [lpe_pos]
  local_position_estimator/7 -> Mux17/1
  local_position_estimator/8 -> Mux17/2
  local_position_estimator/9 -> Mux17/3
  Mux17/1 -> [lpe_vel]
  local_position_estimator/4 -> Mux18/1
  local_position_estimator/5 -> Mux18/2
  local_position_estimator/6 -> Mux18/3
  Mux18/1 -> [gpos_vel]
  local_position_estimator/1 -> [lpe_cov]
  local_position_estimator/2 -> [lpe_health]
  local_position_estimator/3 -> [lpe_states]
  [att_q] -> Quaternion to Euler Angles/1
  Mux19/1 -> Position/1
  Mux20/1 -> Position/2
  Mux21/1 -> Position/3
  Select 19/1 -> Mux21/1  "actual3"
  Select 22/1 -> Mux21/2  "est3"
  Select 21/1 -> Mux20/2  "est2"
  Select 18/1 -> Mux20/1  "actual2"
  Select 20/1 -> Mux19/2  "est1"
  Select 23/1 -> Mux19/1  "actual1"
  [lpe_pos] -> To Workspace1/1, Select 20/1, Select 21/1, Select 22/1
  [lpe_cov] -> Demux5/1
  [xi] -> Select 23/1, Select 18/1, Select 19/1, To Workspace/1
  Mux1/1 -> Velocity/1
  Mux2/1 -> Velocity/2
  Mux3/1 -> Velocity/3
  Select 25/1 -> Mux3/1  "actual3"
  Select 28/1 -> Mux3/2  "est3"
  Select 27/1 -> Mux2/2  "est2"
  Select 24/1 -> Mux2/1  "actual2"
  Select 26/1 -> Mux1/2  "est1"
  Select 29/1 -> Mux1/1  "actual1"
  [lpe_vel] -> To Workspace5/1, Select 28/1, Select 27/1, Select 26/1  "velEst"
  [xiDot] -> To Workspace4/1, Select 25/1, Select 24/1, Select 29/1  "vel"
  Mux4/1 -> Velocity (Global)/1
  Mux5/1 -> Velocity (Global)/2
  Mux22/1 -> Velocity (Global)/3
  Select 31/1 -> Mux22/1  "actual3"
  Select 34/1 -> Mux22/2  "est3"
  Select 33/1 -> Mux5/2  "est2"
  Select 30/1 -> Mux5/1  "actual2"
  Select 32/1 -> Mux4/2  "est1"
  Select 35/1 -> Mux4/1  "actual1"
  [gpos_vel] -> Select 32/1, Select 33/1, Select 34/1
  [xiDot] -> Select 35/1, Select 30/1, Select 31/1
  [accelero] -> local_position_estimator/8
  local_position_estimator/13 -> [lpe_yaw]
  Mux/1 -> [att_nuBody]
  attitude_estimator_q/3 -> Mux/2
  attitude_estimator_q/2 -> Mux/1
  attitude_estimator_q/4 -> Mux/3
  Select 38/1 -> Mux13/2
  Select 37/1 -> Mux15/2
  [att_nuBody] -> Select 38/1, Select 36/1, Select 37/1
  Select 36/1 -> Mux14/2
  Mux23/1 -> [att_xiDDot]
  attitude_estimator_q/7 -> Mux23/2
  attitude_estimator_q/6 -> Mux23/1
  attitude_estimator_q/8 -> Mux23/3
  Mux24/1 -> Acceleration/1
  Mux25/1 -> Acceleration/2
  Mux26/1 -> Acceleration/3
  Select 41/1 -> Mux24/1  "xDDot"
  Select 39/1 -> Mux25/1  "yDDot"
  Select 40/1 -> Mux26/1  "zDDot"
  [accelero] -> Select 39/1, Select 40/1, Select 41/1
  Select 44/1 -> Mux24/2  "xDDotFilt"
  Select 43/1 -> Mux26/2  "zDDotFilt"
  [att_xiDDot] -> Select 43/1, Select 42/1, Select 44/1
  Select 42/1 -> Mux25/2  "yDDotFild"
  attitude_estimator_q/1 -> [att_timestamp]
  [att_q] -> qMeasured/1
  [att_nuBody] -> nuBodyMeasured/1
  xiDDot/1 -> xiDDotMeasured/1, [xiDDot]
  [lpe_pos] -> xiMeasured/1
  [lpe_vel] -> xiDotMeasured/1
  Ground/1 -> attitude_estimator_q/2, attitude_estimator_q/1

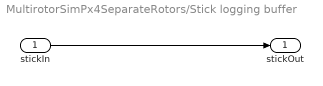
== system MultirotorSimPx4SeparateRotors/Stick logging buffer ==
  stickIn : Inport
  stickOut : Outport
  wires:
  stickIn/1 -> stickOut/1

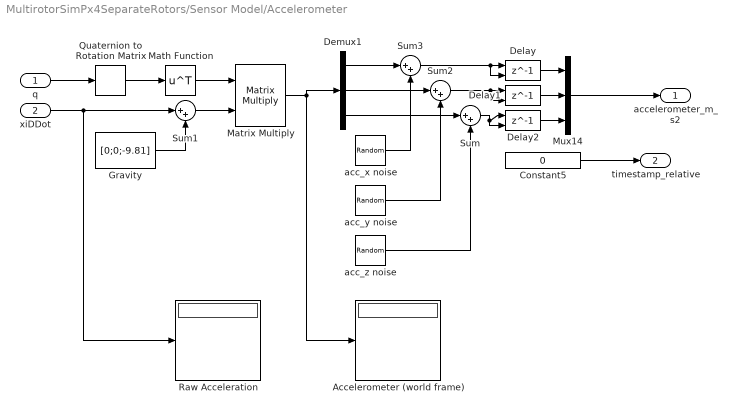
== system MultirotorSimPx4SeparateRotors/Sensor Model/Accelerometer ==
  q : Inport
  xiDDot : Inport  Port=2  Unit=m/s^2
  Accelerometer (world frame) : Display
  Constant5 : Constant  Value=0
  Delay : Delay  DelayLength=1  InitialConditionSource=Input port  SampleTime=1/400
      settings: InputPortMap=u0,p4
  Delay1 : Delay  DelayLength=1  InitialConditionSource=Input port  SampleTime=1/400
      settings: InputPortMap=u0,p4
  Delay2 : Delay  DelayLength=1  InitialConditionSource=Input port  SampleTime=1/400
      settings: InputPortMap=u0,p4
  Demux1 : Demux  Outputs=3
  Gravity : Constant  Value=[0;0;-9.81]
  Math Function : Math  Operator=transpose  SaturateOnIntegerOverflow=on
  Matrix Multiply : Product  Multiplication=Matrix(*)
  Mux14 : Mux  Inputs=3
  Quaternion to Rotation Matrix : QuaternionLibrary/Quaternion to Rotation Matrix
  Raw Acceleration : Display
  Sum{,1..3} (4 alike) : Sum  Inputs=|++
  acc_x noise : RandomNumber  Variance=0.012^2  SampleTime=1/400
  acc_y noise : RandomNumber  Variance=0.012^2  SampleTime=1/400
  acc_z noise : RandomNumber  Variance=0.02^2  SampleTime=1/400
  accelerometer_m_s2 : Outport  Unit=m/s^2  SampleTime=1/400
  timestamp_relative : Outport  Port=2  Unit=µs  SampleTime=1/400
  wires:
  Quaternion to Rotation Matrix/1 -> Math Function/1
  Math Function/1 -> Matrix Multiply/1
  Matrix Multiply/1 -> Accelerometer (world frame)/1, Demux1/1
  Gravity/1 -> Sum1/2
  Sum1/1 -> Matrix Multiply/2
  Mux14/1 -> accelerometer_m_s2/1
  xiDDot/1 -> Raw Acceleration/1, Sum1/1
  q/1 -> Quaternion to Rotation Matrix/1
  Constant5/1 -> timestamp_relative/1
  Demux1/1 -> Sum3/1
  Demux1/2 -> Sum2/1
  Demux1/3 -> Sum/1
  Sum/1 -> Delay2/2, Delay2/1
  acc_z noise/1 -> Sum/2
  Sum2/1 -> Delay1/2, Delay1/1
  Sum3/1 -> Delay/2, Delay/1
  acc_y noise/1 -> Sum2/2
  acc_x noise/1 -> Sum3/2
  Delay/1 -> Mux14/1
  Delay1/1 -> Mux14/2
  Delay2/1 -> Mux14/3

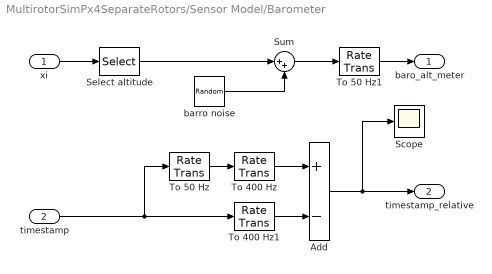
== system MultirotorSimPx4SeparateRotors/Sensor Model/Barometer ==
  xi : Inport  Unit=m
  timestamp : Inport  Port=2  Unit=µs
  Add : Sum  Inputs=+-
  Scope : Scope
  Select altitude : Selector  InputPortWidth=3  IndexOptions=Index vector (dialog)  Indices=3  OutputSizes=1
  Sum : Sum  Inputs=|++
  To 400 Hz : RateTransition  Deterministic=off  OutPortSampleTime=1/250
  To 400 Hz1 : RateTransition  OutPortSampleTime=1/400
  To 50 Hz : RateTransition  OutPortSampleTime=1/50
  To 50 Hz1 : RateTransition  OutPortSampleTime=1/50
  barro noise : RandomNumber  Variance=1/3^2  SampleTime=0.01
  baro_alt_meter : Outport  Unit=m  SampleTime=1/400
  timestamp_relative : Outport  Port=2  Unit=µs
  wires:
  barro noise/1 -> Sum/2
  Sum/1 -> To 50 Hz1/1
  xi/1 -> Select altitude/1
  Select altitude/1 -> Sum/1
  Add/1 -> timestamp_relative/1, Scope/1
  To 400 Hz1/1 -> Add/2
  To 50 Hz/1 -> To 400 Hz/1
  To 400 Hz/1 -> Add/1
  timestamp/1 -> To 50 Hz/1, To 400 Hz1/1
  To 50 Hz1/1 -> baro_alt_meter/1

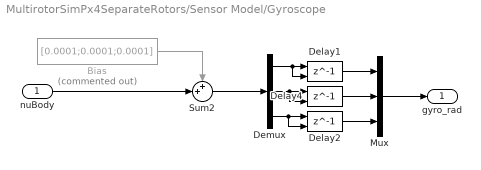
== system MultirotorSimPx4SeparateRotors/Sensor Model/Gyroscope ==
  nuBody : Inport  Unit=rad/s
  Bias : Constant  Commented=on  Value=[0.0001;0.0001;0.0001]
  Delay1 : Delay  DelayLength=1  InitialConditionSource=Input port  SampleTime=1/400
      settings: InputPortMap=u0,p4
  Delay2 : Delay  DelayLength=1  InitialConditionSource=Input port  SampleTime=1/400
      settings: InputPortMap=u0,p4
  Delay4 : Delay  DelayLength=1  InitialConditionSource=Input port  SampleTime=1/400
      settings: InputPortMap=u0,p4
  Demux : Demux  Outputs=3
  Mux : Mux  Inputs=3
  Sum2 : Sum  Inputs=++|
  gyro_rad : Outport  Unit=rad/s  SampleTime=1/400
  wires:
  Sum2/1 -> Demux/1
  Mux/1 -> gyro_rad/1
  Bias/1 -> Sum2/1
  nuBody/1 -> Sum2/2
  Delay4/1 -> Mux/2
  Delay2/1 -> Mux/3
  Delay1/1 -> Mux/1
  Demux/1 -> Delay1/2, Delay1/1
  Demux/2 -> Delay4/2, Delay4/1
  Demux/3 -> Delay2/2, Delay2/1

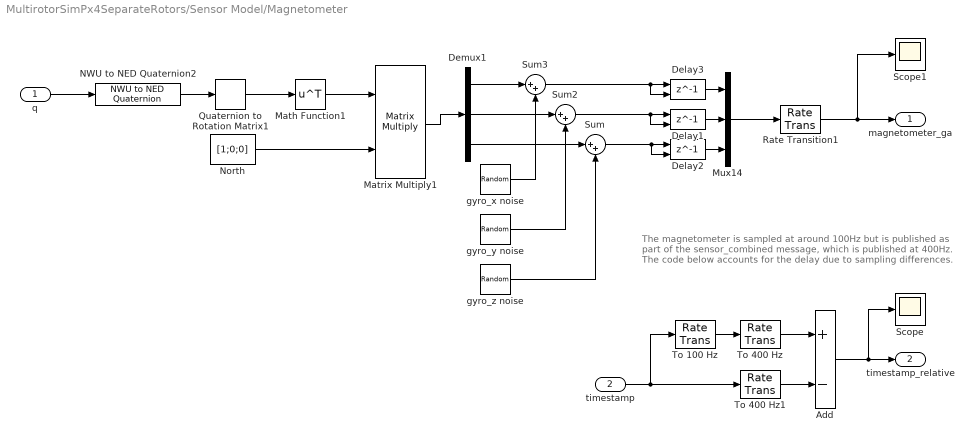
== system MultirotorSimPx4SeparateRotors/Sensor Model/Magnetometer ==
  note: The magnetometer is sampled at around 100Hz but is published
      | as part of the sensor_combined message, which is published at
      | 400Hz. The code below accounts for the delay due to sampling
      | differences.
  q : Inport
  timestamp : Inport  Port=2
  Add : Sum  Inputs=+-
  Delay1 : Delay  DelayLength=1  InitialConditionSource=Input port  SampleTime=1/100
      settings: InputPortMap=u0,p4
  Delay2 : Delay  DelayLength=1  InitialConditionSource=Input port  SampleTime=1/100
      settings: InputPortMap=u0,p4
  Delay3 : Delay  DelayLength=1  InitialConditionSource=Input port  SampleTime=1/100
      settings: InputPortMap=u0,p4
  Demux1 : Demux  Outputs=3
  Math Function1 : Math  Operator=transpose  SaturateOnIntegerOverflow=on
  Matrix Multiply1 : Product  Multiplication=Matrix(*)
  Mux14 : Mux  Inputs=3
  NWU to NED Quaternion2 : Px4Library/NWU to NED Quaternion
  North : Constant  Value=[1;0;0]
  Quaternion to Rotation Matrix1 : QuaternionLibrary/Quaternion to Rotation Matrix
  Rate Transition1 : RateTransition  Deterministic=off  OutPortSampleTime=1/100
  Scope : Scope
  Scope1 : Scope
  Sum : Sum  Inputs=|++
  Sum2 : Sum  Inputs=|++
  Sum3 : Sum  Inputs=|++
  To 100 Hz : RateTransition  OutPortSampleTime=1/100
  To 400 Hz : RateTransition  Deterministic=off  OutPortSampleTime=1/250
  To 400 Hz1 : RateTransition  OutPortSampleTime=1/400
  gyro_x noise : RandomNumber  Variance=0.001^2  SampleTime=1/400
  gyro_y noise : RandomNumber  Variance=0.001^2  SampleTime=1/400
  gyro_z noise : RandomNumber  Variance=0.001^2  SampleTime=1/400
  magnetometer_ga : Outport  Unit=G  SampleTime=1/250
  timestamp_relative : Outport  Port=2  Unit=µs  SampleTime=1/250
  wires:
  NWU to NED Quaternion2/1 -> Quaternion to Rotation Matrix1/1
  Quaternion to Rotation Matrix1/1 -> Math Function1/1
  q/1 -> NWU to NED Quaternion2/1
  North/1 -> Matrix Multiply1/2
  Math Function1/1 -> Matrix Multiply1/1
  Add/1 -> timestamp_relative/1, Scope/1
  Matrix Multiply1/1 -> Demux1/1
  Demux1/1 -> Sum3/1
  Demux1/2 -> Sum2/1
  Demux1/3 -> Sum/1
  Sum/1 -> Delay2/2, Delay2/1
  gyro_z noise/1 -> Sum/2
  Sum2/1 -> Delay1/2, Delay1/1
  gyro_y noise/1 -> Sum2/2
  gyro_x noise/1 -> Sum3/2
  Mux14/1 -> Rate Transition1/1
  To 400 Hz1/1 -> Add/2
  To 100 Hz/1 -> To 400 Hz/1
  To 400 Hz/1 -> Add/1
  Rate Transition1/1 -> Scope1/1, magnetometer_ga/1
  timestamp/1 -> To 100 Hz/1, To 400 Hz1/1
  Delay3/1 -> Mux14/1
  Sum3/1 -> Delay3/2, Delay3/1
  Delay1/1 -> Mux14/2
  Delay2/1 -> Mux14/3

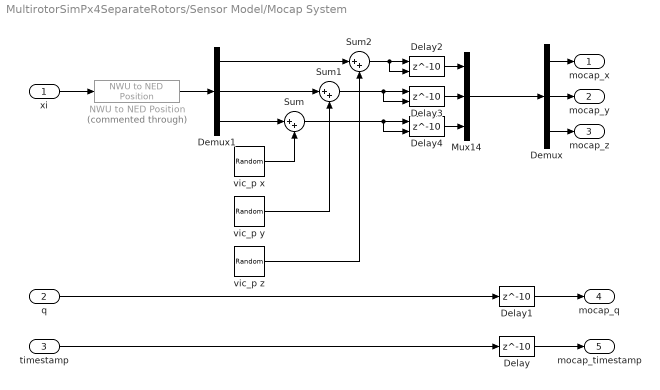
== system MultirotorSimPx4SeparateRotors/Sensor Model/Mocap System ==
  xi : Inport
  q : Inport  Port=2
  timestamp : Inport  Port=3
  Delay : Delay  DelayLength=10  SampleTime=1/100
  Delay1 : Delay  DelayLength=10  SampleTime=1/100
  Delay2 : Delay  DelayLength=10  InitialConditionSource=Input port  SampleTime=1/100
      settings: InputPortMap=u0,p4
  Delay3 : Delay  DelayLength=10  InitialConditionSource=Input port  SampleTime=1/100
      settings: InputPortMap=u0,p4
  Delay4 : Delay  DelayLength=10  InitialConditionSource=Input port  SampleTime=1/100
      settings: InputPortMap=u0,p4
  Demux : Demux  Outputs=3
  Demux1 : Demux  Outputs=3
  Mux14 : Mux  Inputs=3
  NWU to NED Position : Px4Library/NWU to NED Position  Commented=through
  Sum : Sum  Inputs=|++
  Sum1 : Sum  Inputs=|++
  Sum2 : Sum  Inputs=|++
  vic_p x : RandomNumber  Variance=0.001^2  SampleTime=0.01
  vic_p y : RandomNumber  Variance=0.001^2  SampleTime=0.01
  vic_p z : RandomNumber  Variance=0.001^2  SampleTime=0.01
  mocap_x : Outport
  mocap_y : Outport  Port=2
  mocap_z : Outport  Port=3
  mocap_q : Outport  Port=4
  mocap_timestamp : Outport  Port=5
  wires:
  q/1 -> Delay1/1
  timestamp/1 -> Delay/1
  Delay/1 -> mocap_timestamp/1
  Delay1/1 -> mocap_q/1
  Demux1/1 -> Sum2/1
  Demux1/2 -> Sum1/1
  NWU to NED Position/1 -> Demux1/1
  Demux1/3 -> Sum/1
  Sum/1 -> Delay4/2, Delay4/1
  vic_p x/1 -> Sum/2
  Sum1/1 -> Delay3/2, Delay3/1
  Sum2/1 -> Delay2/2, Delay2/1
  vic_p y/1 -> Sum1/2
  vic_p z/1 -> Sum2/2
  xi/1 -> NWU to NED Position/1
  Demux/3 -> mocap_z/1
  Demux/2 -> mocap_y/1
  Demux/1 -> mocap_x/1
  Mux14/1 -> Demux/1
  Delay2/1 -> Mux14/1
  Delay3/1 -> Mux14/2
  Delay4/1 -> Mux14/3

== matlab function MultirotorSimPx4SeparateRotors/Quadrotor Quaternion Model/Equations of motion ==
  data: VBody input; VBodyDot output; nuBody input; Q input; TBody input size=3; tauBody input size=3; F_D input size=3; M_D input size=3; nuBodyDot output; Uav parameter; xiDDot output
function [VBodyDot, nuBodyDot, xiDDot] = QuadrotorQuaternionModel(...
    VBody, nuBody, Q, TBody, tauBody, F_D, M_D, Uav)
%#codegen

%% Rotation matrices

%% Moments and Forces
% Body frame accelerations
VBodyDot  = (1/Uav.M) * (Q'*Uav.G + TBody - cross(nuBody, Uav.M*VBody) - F_D);
nuBodyDot = Uav.I \ (tauBody - cross(nuBody, Uav.I*nuBody) - M_D);

% Inertial frame accelerations
xiDDot = (1/Uav.M)*(Uav.G + Q*(TBody - F_D));
% etaDDot = WInvertDot*nuBody + WInvert*nuBodyDot;

% Check centripetal force in inertial frame
% F_C = R*cross(nuBody,m*VBody);
end

== matlab function MultirotorSimPx4SeparateRotors/Compute Sph ==
  data: V_appBody input; azimuth output; elevation output; radius output
function [azimuth, elevation, radius] = computeSph(V_appBody)
%#codegen

% Convert from polar to spherical coordinates
[ azimuth, elevation, radius ] = cart2sph( V_appBody(1), V_appBody(2), V_appBody(3) );

== matlab function MultirotorSimPx4SeparateRotors/Applied wind speed/Relative velocity ==
  data: nuBody input; Uav parameter; VMotorRelBody output size=[3,4]
function VMotorRelBody = relativeMotorVelocity( nuBody , Uav )
%#codegen
assert(Uav.N_ROTORS < 16);

VMotorRelBody = zeros(3, 4);
% VMotorRelMotor = zeros(3, Uav.N_ROTORS);

for i = 1:length( Uav.N_ROTORS )
    VMotorRelBody(:,i) = cross( nuBody, Uav.L_VEC(:,i) );
    % VMotorRelMotor(:,i) = Uav.R_MOTOR_TO_BODY(:,:,i)' * VMotorRelBody;
end

== matlab function MultirotorSimPx4SeparateRotors/Applied wind speed/Compute V_app2 ==
  data: Q input; UBody output; U input size=3
function UBody = computeUBody(Q, U)
%#codegen

% Rotation matrix from Wind frame to Inertial frame 
R_U = [1, 0,  0;
       0, 1,  0;
       0, 0, -1];
   
UBody = Q' * R_U * U;
